simulink subsystem "sort2"  (R2021b)
settings: Solver=VariableStepAuto  StartTime=0.0  StopTime=10.0  RelTol=1e-3
settings Model: Creator=dileepan  LastModifiedBy=dileepan

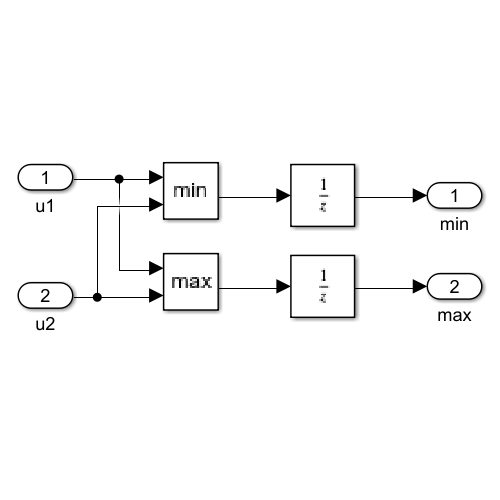
[thumbnail: Simulink's stored preview of the top-level diagram]
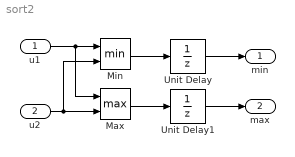
== system sort2 ==
  u1 : Inport
  u2 : Inport  Port=2
  Max : MinMax  Function=max  Inputs=2
  Min : MinMax  Inputs=2
  Unit Delay : UnitDelay  SampleTime=-1  HasFrameUpgradeWarning=on
  Unit Delay1 : UnitDelay  SampleTime=-1  HasFrameUpgradeWarning=on
  min : Outport
  max : Outport  Port=2
  wires:
  Min/1 -> Unit Delay/1
  u2/1 -> Max/2, Min/2
  Unit Delay1/1 -> max/1
  Max/1 -> Unit Delay1/1
  Unit Delay/1 -> min/1
  u1/1 -> Max/1, Min/1
